simulink model "untitled"  (R2019a)
settings: Solver=VariableStepAuto  StartTime=0.0  StopTime=10.0  RelTol=1e-3
settings Model: Creator=PC  LastModifiedBy=PC

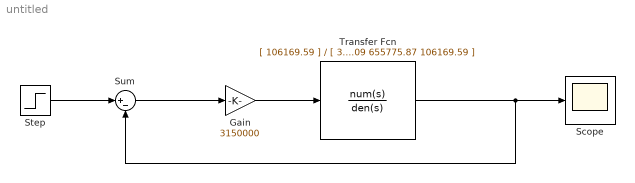
== system untitled ==
  Gain : Gain  Gain=3150000
  Scope : Scope
  Step : Step  SampleTime=0
  Sum : Sum  Inputs=|+-
  Transfer Fcn : TransferFcn  Numerator=[ 106169.59 ]  Denominator=[ 3.09 655775.87 106169.59 ]
  wires:
  Transfer Fcn/1 -> Sum/2, Scope/1
  Gain/1 -> Transfer Fcn/1
  Step/1 -> Sum/1
  Sum/1 -> Gain/1
